simulink model "Fuel_system"  (R2017b)
settings: Solver=ode1  StartTime=0.0  StopTime=inf  FixedStep=0.001  RelTol=1e-3
model workspace (MAT data in the model file):
  sample_time = Simulink.Parameter
  sample_time.DataType = 'auto'
  sample_time.Dimensions = [0 0]
libraries: SIPLib x1
settings Model: Creator=pavel.dushkin  LastModifiedBy=pavel.dushkin
settings DataIOCC: SaveFormat=StructureWithTime  SaveState=on  ReturnWorkspaceOutputs=on
settings OptimizationCC: OptimizeBlockIOStorage=off  BufferReuse=off  GlobalBufferReuse=off  ExpressionFolding=off  LocalBlockOutputs=off  OptimizeDataStoreBuffers=off  BusAssignmentInplaceUpdate=off
settings DebuggingCC: ReadBeforeWriteMsg=DisableAll  WriteAfterWriteMsg=DisableAll  WriteAfterReadMsg=DisableAll  MultiTaskDSMMsg=none
settings ModelReferenceCC: UpdateModelReferenceTargets=IfOutOfDate

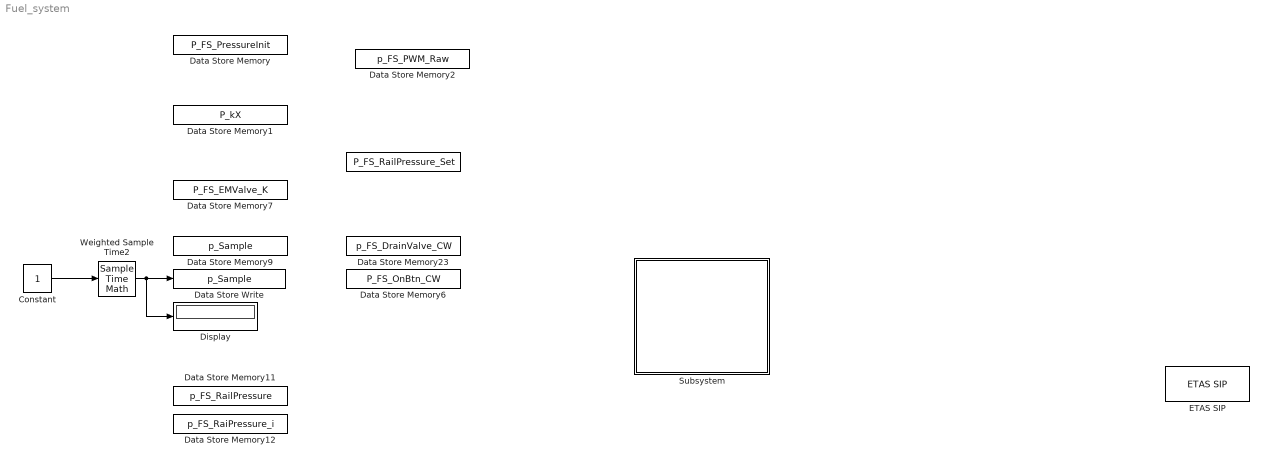
== system Fuel_system ==
  " " : DataStoreMemory  DataStoreName=P_FS_RailPressure_Set  ReadBeforeWriteMsg=warning  WriteAfterWriteMsg=warning  WriteAfterReadMsg=warning  ShowAdditionalParam=off  OutDataTypeStr=double
  Constant : Constant  OutDataTypeStr=double
  Data Store Memory : DataStoreMemory  DataStoreName=P_FS_PressureInit  ReadBeforeWriteMsg=warning  WriteAfterWriteMsg=warning  WriteAfterReadMsg=warning  ShowAdditionalParam=off  OutDataTypeStr=double
  Data Store Memory1 : DataStoreMemory  DataStoreName=P_kX  ReadBeforeWriteMsg=warning  WriteAfterWriteMsg=warning  WriteAfterReadMsg=warning  ShowAdditionalParam=off  OutDataTypeStr=double
  Data Store Memory11 : DataStoreMemory  DataStoreName=p_FS_RailPressure  ReadBeforeWriteMsg=warning  WriteAfterWriteMsg=warning  WriteAfterReadMsg=warning  ShowAdditionalParam=off  OutDataTypeStr=double
  Data Store Memory12 : DataStoreMemory  DataStoreName=p_FS_RaiPressure_i  ReadBeforeWriteMsg=warning  WriteAfterWriteMsg=warning  WriteAfterReadMsg=warning  ShowAdditionalParam=off  OutDataTypeStr=double
  Data Store Memory2 : DataStoreMemory  DataStoreName=p_FS_PWM_Raw  ReadBeforeWriteMsg=warning  WriteAfterWriteMsg=warning  WriteAfterReadMsg=warning  ShowAdditionalParam=off  OutDataTypeStr=double
  Data Store Memory23 : DataStoreMemory  DataStoreName=p_FS_DrainValve_CW  ReadBeforeWriteMsg=warning  WriteAfterWriteMsg=warning  WriteAfterReadMsg=warning  ShowAdditionalParam=off  OutDataTypeStr=double
  Data Store Memory6 : DataStoreMemory  DataStoreName=P_FS_OnBtn_CW  ReadBeforeWriteMsg=warning  WriteAfterWriteMsg=warning  WriteAfterReadMsg=warning  ShowAdditionalParam=off  OutDataTypeStr=double
  Data Store Memory7 : DataStoreMemory  DataStoreName=P_FS_EMValve_K  ReadBeforeWriteMsg=warning  WriteAfterWriteMsg=warning  WriteAfterReadMsg=warning  ShowAdditionalParam=off  OutDataTypeStr=double
  Data Store Memory9 : DataStoreMemory  DataStoreName=p_Sample  ReadBeforeWriteMsg=warning  WriteAfterWriteMsg=warning  WriteAfterReadMsg=warning  ShowAdditionalParam=off  OutDataTypeStr=double
  Data Store Write : DataStoreWrite  DataStoreName=p_Sample
  Display : Display
  ETAS SIP : SIPLib/ETAS SIP
  Subsystem : Subsystem
  Weighted Sample Time2 : SampleTimeMath  TsampMathOp=Ts Only
  wires:
  Weighted Sample Time2/1 -> Display/1, Data Store Write/1
  Constant/1 -> Weighted Sample Time2/1

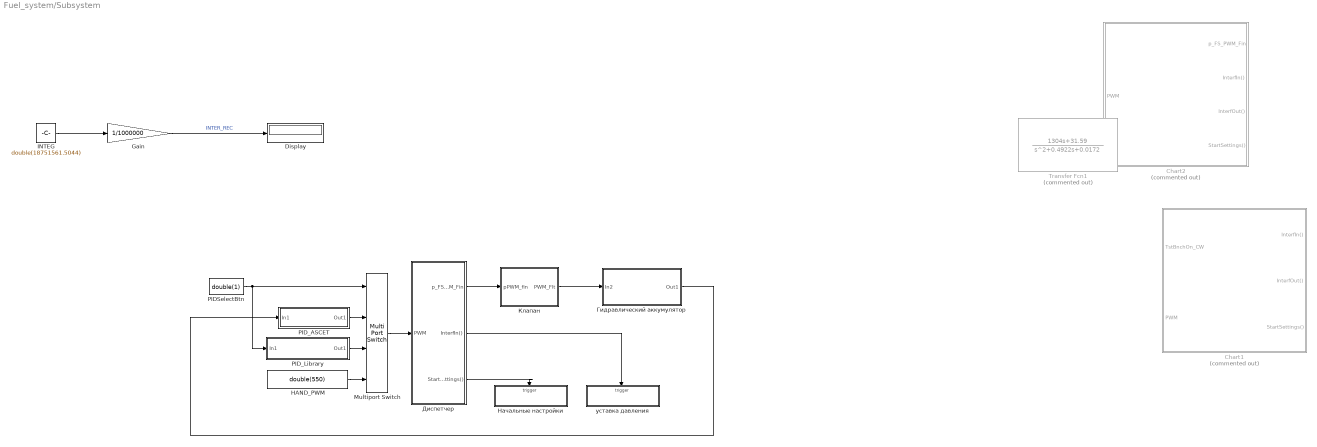
== system Fuel_system/Subsystem ==
  Chart1 : Stateflow chart  Commented=on  TreatAsAtomicUnit=on
  Chart2 : Stateflow chart  Commented=on  TreatAsAtomicUnit=on
  Display : Display
  Gain : Gain  Gain=1/1000000
  HAND_PWM : Constant  Value=double(550)  OutDataTypeStr=single
  INTEG : Constant  Value=double(18751561.5044)
  Multiport Switch : MultiPortSwitch
  PIDSelectBtn : Constant  Value=double(1)  OutDataTypeStr=uint8
  PID_ASCET : Subsystem
  PID_Library : Subsystem
  Transfer Fcn1 : TransferFcn  Commented=on  Numerator=[1304 31.59]  Denominator=[1 0.4922 0.0172]
  Гидравлический аккумулятор : Subsystem
  Диспетчер : Stateflow chart  TreatAsAtomicUnit=on
  Клапан : Subsystem
  Начальные настройки : Subsystem
  уставка давления : Subsystem
  wires:
  PID_ASCET/1(Out1) -> Multiport Switch/2
  HAND_PWM/1 -> Multiport Switch/4
  PID_Library/1(Out1) -> Multiport Switch/3
  PIDSelectBtn/1 -> Multiport Switch/1, PID_Library/1(In1)
  Диспетчер/3(StartSettings()) -> Начальные настройки/Trigger
  Multiport Switch/1 -> Диспетчер/1(PWM)
  Диспетчер/2(InterfIn()) -> уставка давления/Trigger
  Гидравлический аккумулятор/1(Out1) -> PID_ASCET/1(In1)
  INTEG/1 -> Gain/1
  Gain/1 -> Display/1  "INTER_REC"
  Диспетчер/1(p_FS_PWM_Fin) -> Клапан/1(pPWM_fin)
  Клапан/1(PWM_Flt) -> Гидравлический аккумулятор/1(In2)

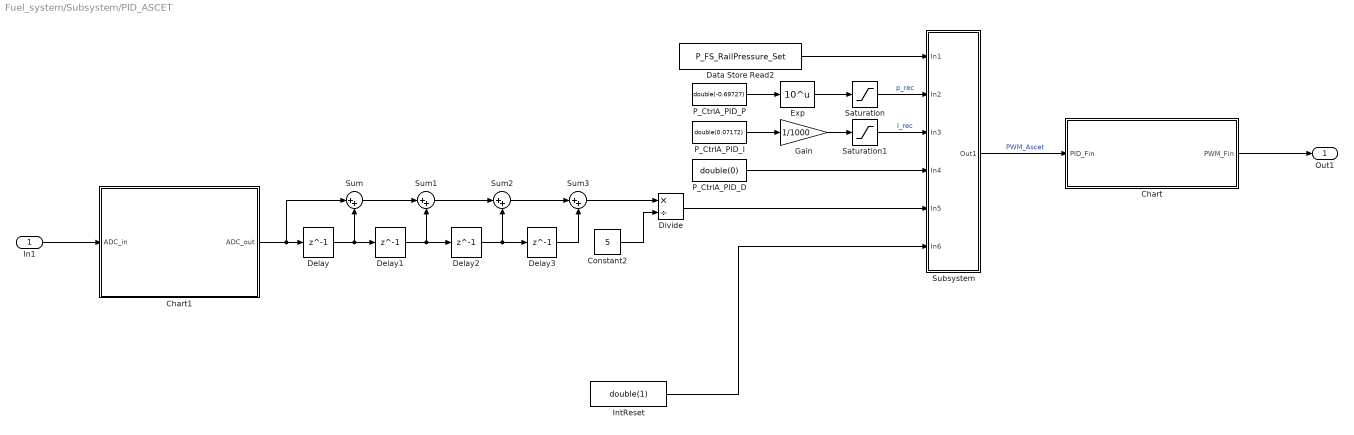
== system Fuel_system/Subsystem/PID_ASCET ==
  In1 : Inport
  Chart : Stateflow chart  TreatAsAtomicUnit=on
  Chart1 : Stateflow chart  TreatAsAtomicUnit=on
  Constant2 : Constant  Value=5
  Data Store Read2 : DataStoreRead  DataStoreName=P_FS_RailPressure_Set
  Delay{,1..3} (4 alike) : Delay  DelayLength=1  InitialCondition=0
  Divide : Product  Inputs=*/  OutDataTypeStr=single
  Exp : Math  Operator=10^u  OutputSignalType=real  SaturateOnIntegerOverflow=on
  Gain : Gain  Gain=1/1000
  IntReset : Constant  Value=double(1)  OutDataTypeStr=single
  P_CtrlA_PID_D : Constant  Value=double(0)  OutDataTypeStr=single
  P_CtrlA_PID_I : Constant  Value=double(0.07172)  OutDataTypeStr=single
  P_CtrlA_PID_P : Constant  Value=double(-0.69727)  OutDataTypeStr=single
  Saturation : Saturate  UpperLimit=inf  LowerLimit=0
  Saturation1 : Saturate  UpperLimit=inf  LowerLimit=0.01/1000
  Subsystem : Subsystem
  Sum{,1..3} (4 alike) : Sum  Inputs=|++
  Out1 : Outport
  wires:
  P_CtrlA_PID_D/1 -> Subsystem/4(In4)
  P_CtrlA_PID_P/1 -> Exp/1
  P_CtrlA_PID_I/1 -> Gain/1
  Subsystem/1(Out1) -> Chart/1(PID_Fin)  "PWM_Ascet"
  Data Store Read2/1 -> Subsystem/1(In1)
  Divide/1 -> Subsystem/5(In5)
  IntReset/1 -> Subsystem/6(In6)
  Chart1/1(ADC_out) -> Sum/1, Delay/1
  Delay/1 -> Sum/2, Delay1/1
  Delay1/1 -> Sum1/2, Delay2/1
  Delay2/1 -> Sum2/2, Delay3/1
  Delay3/1 -> Sum3/2
  Sum/1 -> Sum1/1
  Sum1/1 -> Sum2/1
  Sum2/1 -> Sum3/1
  Sum3/1 -> Divide/1
  Constant2/1 -> Divide/2
  Chart/1(PWM_Fin) -> Out1/1
  Gain/1 -> Saturation1/1
  Exp/1 -> Saturation/1
  In1/1 -> Chart1/1(ADC_in)
  Saturation/1 -> Subsystem/2(In2)  "p_rec"
  Saturation1/1 -> Subsystem/3(In3)  "I_rec"

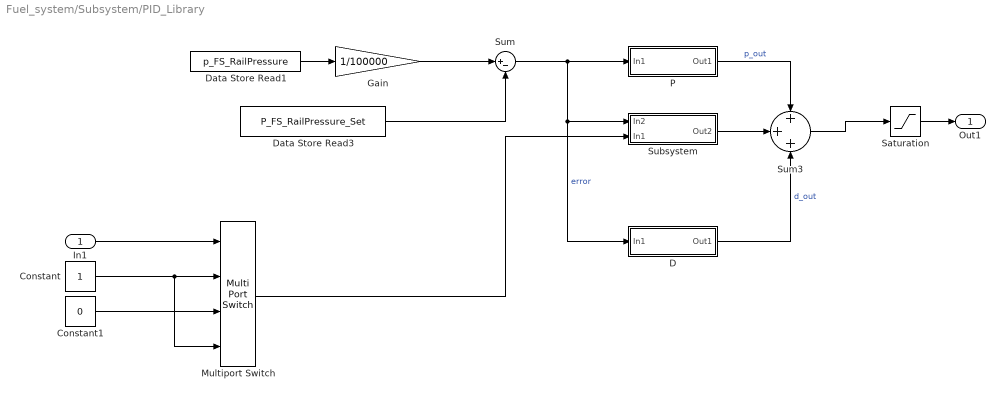
== system Fuel_system/Subsystem/PID_Library ==
  In1 : Inport
  Constant : Constant
  Constant1 : Constant  Value=0
  D : Subsystem
  Data Store Read1 : DataStoreRead  DataStoreName=p_FS_RailPressure
  Data Store Read3 : DataStoreRead  DataStoreName=P_FS_RailPressure_Set
  Gain : Gain  Gain=1/100000
  Multiport Switch : MultiPortSwitch
  P : Subsystem
  Saturation : Saturate  UpperLimit=50  LowerLimit=30
  Subsystem : Subsystem
  Sum : Sum  Inputs=|+-
  Sum3 : Sum  Inputs=+++
  Out1 : Outport
  wires:
  Sum3/1 -> Saturation/1
  P/1(Out1) -> Sum3/1  "p_out"
  Data Store Read1/1 -> Gain/1
  Saturation/1 -> Out1/1
  Sum/1 -> Subsystem/1(In2), D/1(In1), P/1(In1)  "error"
  D/1(Out1) -> Sum3/3  "d_out"
  Subsystem/1(Out2) -> Sum3/2
  In1/1 -> Multiport Switch/1
  Constant/1 -> Multiport Switch/4, Multiport Switch/2
  Multiport Switch/1 -> Subsystem/2(In1)
  Constant1/1 -> Multiport Switch/3
  Data Store Read3/1 -> Sum/2
  Gain/1 -> Sum/1

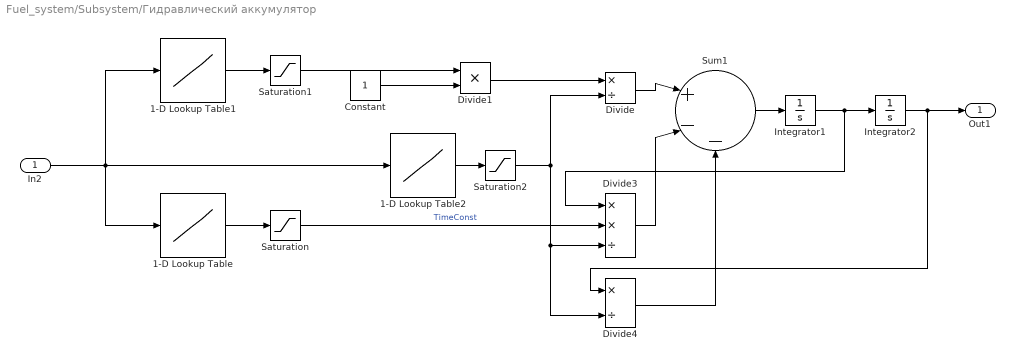
== system Fuel_system/Subsystem/Гидравлический аккумулятор ==
  In2 : Inport
  1-D Lookup Table : Lookup_n-D  NumberOfTableDimensions=1  BreakpointsForDimension1=[100 450 500 550]  Table=[0.03 0.03 1.55 9]  InternalRulePriority=Speed  RndMeth=Simplest  InputSameDT=on
  1-D Lookup Table1 : Lookup_n-D  NumberOfTableDimensions=1  BreakpointsForDimension1=[100 450 500 550]  Table=[3500 2500 1950 925]  InternalRulePriority=Speed  RndMeth=Simplest  InputSameDT=on
  1-D Lookup Table2 : Lookup_n-D  NumberOfTableDimensions=1  BreakpointsForDimension1=[100 450 500 550]  Table=[0.2 0.5 1 1]  InternalRulePriority=Speed  RndMeth=Simplest  InputSameDT=on
  Constant : Constant
  Divide : Product  Inputs=*/  OutDataTypeStr=single
  Divide1 : Product  Inputs=**  OutDataTypeStr=single
  Divide3 : Product  Inputs=**/
  Divide4 : Product  Inputs=*/
  Integrator1 : Integrator
  Integrator2 : Integrator
  Saturation : Saturate  UpperLimit=inf  LowerLimit=0.01
  Saturation1 : Saturate  UpperLimit=5000  LowerLimit=0
  Saturation2 : Saturate  UpperLimit=inf  LowerLimit=0.1
  Sum1 : Sum  Inputs=|+--  AccumDataTypeStr=single
  Out1 : Outport
  wires:
  Integrator2/1 -> Out1/1, Divide4/1
  Divide/1 -> Sum1/1
  Sum1/1 -> Integrator1/1
  Integrator1/1 -> Divide3/1, Integrator2/1
  1-D Lookup Table2/1 -> Saturation2/1
  Divide4/1 -> Sum1/3
  Divide3/1 -> Sum1/2
  1-D Lookup Table/1 -> Saturation/1
  1-D Lookup Table1/1 -> Saturation1/1
  Constant/1 -> Divide1/2
  Saturation1/1 -> Divide1/1
  Saturation/1 -> Divide3/2  "TimeConst"
  In2/1 -> 1-D Lookup Table2/1, 1-D Lookup Table/1, 1-D Lookup Table1/1
  Saturation2/1 -> Divide/2, Divide4/2, Divide3/3
  Divide1/1 -> Divide/1

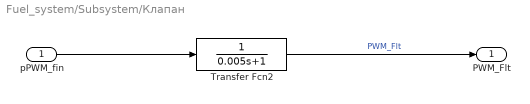
== system Fuel_system/Subsystem/Клапан ==
  pPWM_fin : Inport
  Transfer Fcn2 : TransferFcn  Denominator=[0.005 1]
  PWM_Flt : Outport
  wires:
  pPWM_fin/1 -> Transfer Fcn2/1
  Transfer Fcn2/1 -> PWM_Flt/1  "PWM_Flt"

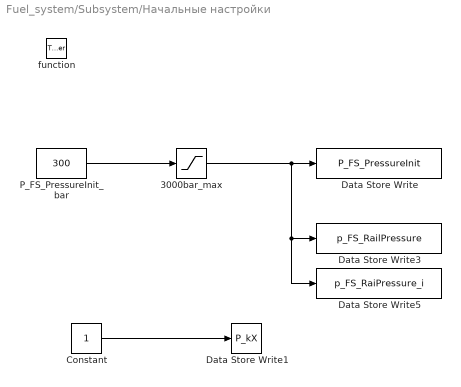
== system Fuel_system/Subsystem/Начальные настройки ==
  function : TriggerPort  TriggerType=function-call  VariantControl=(inherit)
  3000bar_max : Saturate  UpperLimit=3000  LowerLimit=0
  Constant : Constant
  Data Store Write : DataStoreWrite  DataStoreName=P_FS_PressureInit
  Data Store Write1 : DataStoreWrite  DataStoreName=P_kX
  Data Store Write3 : DataStoreWrite  DataStoreName=p_FS_RailPressure
  Data Store Write5 : DataStoreWrite  DataStoreName=p_FS_RaiPressure_i
  P_FS_PressureInit_bar : Constant  Value=300  OutDataTypeStr=double
  wires:
  3000bar_max/1 -> Data Store Write5/1, Data Store Write3/1, Data Store Write/1
  P_FS_PressureInit_bar/1 -> 3000bar_max/1
  Constant/1 -> Data Store Write1/1

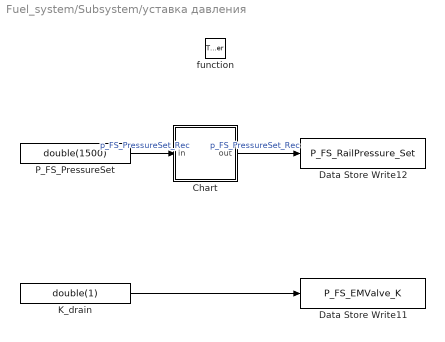
== system Fuel_system/Subsystem/уставка давления ==
  function : TriggerPort  TriggerType=function-call  VariantControl=(inherit)
  Chart : Stateflow chart  TreatAsAtomicUnit=on
  Data Store Write11 : DataStoreWrite  DataStoreName=P_FS_EMValve_K
  Data Store Write12 : DataStoreWrite  DataStoreName=P_FS_RailPressure_Set
  K_drain : Constant  Value=double(1)  OutDataTypeStr=double
  P_FS_PressureSet : Constant  Value=double(1500)  OutDataTypeStr=double
  wires:
  K_drain/1 -> Data Store Write11/1
  Chart/1(out) -> Data Store Write12/1  "p_FS_PressureSet_Rec"
  P_FS_PressureSet/1 -> Chart/1(in)  "p_FS_PressureSet_Rec"

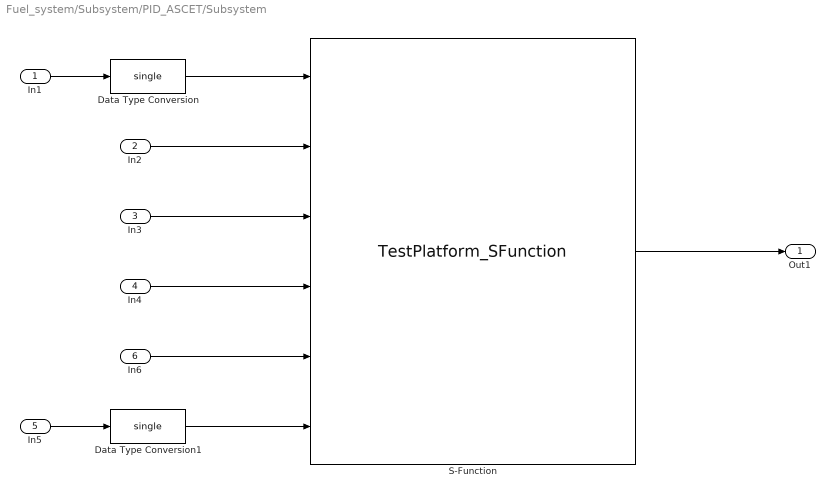
== system Fuel_system/Subsystem/PID_ASCET/Subsystem ==
  In1 : Inport
  In2 : Inport  Port=2
  In3 : Inport  Port=3
  In4 : Inport  Port=4
  In5 : Inport  Port=5
  In6 : Inport  Port=6
  Data Type Conversion : DataTypeConversion  OutDataTypeStr=single
  Data Type Conversion1 : DataTypeConversion  OutDataTypeStr=single
  S-Function : S-Function  InitFcn=clear TestPlatform_SFunction  FunctionName=TestPlatform_SFunction  SFunctionDeploymentMode=off  EnableBusSupport=off
      mask Display:
      | disp('TestPlatform_SFunction')
      | port_label('output',1,'components.InpOut.PWM')
      | port_label('input',1,'components.PID.PressSet')
      | port_label('input',2,'components.PID.qP')
      | port_label('input',3,'components.PID.qI')
      | port_label('input',4,'components.PID.qD')
      | port_label('input',5,'components.PID.I_reset')
      | port_label('input',6,'components.InpOut.MeasuredPressure')
  Out1 : Outport
  wires:
  In1/1 -> Data Type Conversion/1
  In5/1 -> Data Type Conversion1/1
  Data Type Conversion/1 -> S-Function/1
  In2/1 -> S-Function/2
  In3/1 -> S-Function/3
  In4/1 -> S-Function/4
  In6/1 -> S-Function/5
  Data Type Conversion1/1 -> S-Function/6
  S-Function/1 -> Out1/1

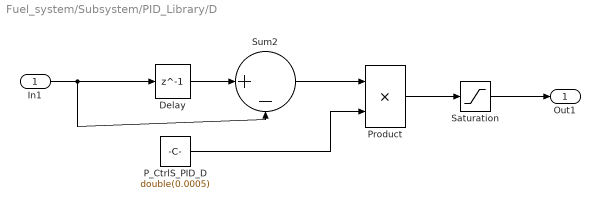
== system Fuel_system/Subsystem/PID_Library/D ==
  In1 : Inport
  Delay : Delay  DelayLength=1
  P_CtrlS_PID_D : Constant  Value=double(0.0005)
  Product : Product
  Saturation : Saturate  UpperLimit=100  LowerLimit=-100
  Sum2 : Sum  Inputs=|+-
  Out1 : Outport
  wires:
  Sum2/1 -> Product/1
  Saturation/1 -> Out1/1
  In1/1 -> Sum2/2, Delay/1
  P_CtrlS_PID_D/1 -> Product/2
  Product/1 -> Saturation/1
  Delay/1 -> Sum2/1

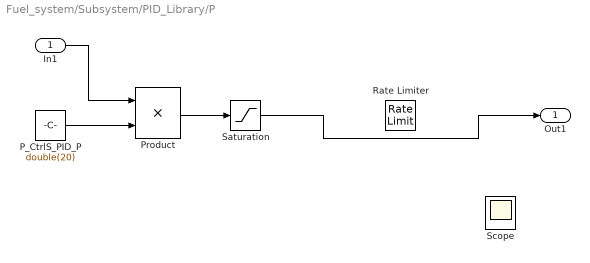
== system Fuel_system/Subsystem/PID_Library/P ==
  In1 : Inport
  P_CtrlS_PID_P : Constant  Value=double(20)
  Product : Product
  Rate Limiter : RateLimiter  RisingSlewLimit=5  FallingSlewLimit=-5  SampleTimeMode=inherited
  Saturation : Saturate  UpperLimit=100  LowerLimit=0
  Scope : Scope  NumInputPorts=2
  Out1 : Outport
  wires:
  In1/1 -> Product/1
  Product/1 -> Saturation/1
  P_CtrlS_PID_P/1 -> Product/2
  Saturation/1 -> Out1/1

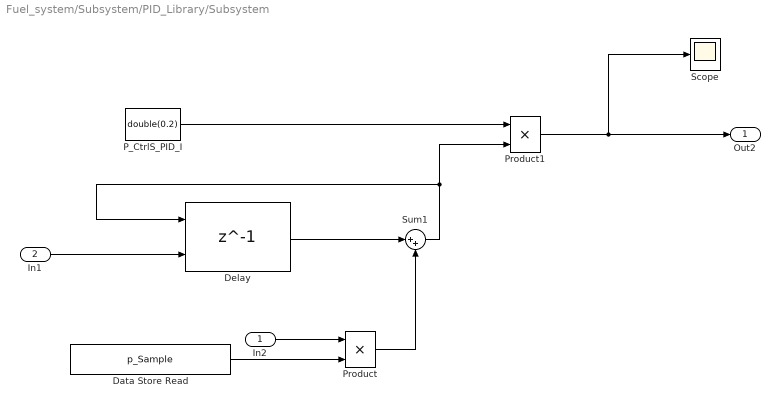
== system Fuel_system/Subsystem/PID_Library/Subsystem ==
  In2 : Inport
  In1 : Inport  Port=2
  Data Store Read : DataStoreRead  DataStoreName=p_Sample
  Delay : Delay  DelayLength=1  ExternalReset=Level
      settings: InputPortMap=u0,r5
  P_CtrlS_PID_I : Constant  Value=double(0.2)
  Product : Product
  Product1 : Product
  Scope : Scope
  Sum1 : Sum  Inputs=|++
  Out2 : Outport
  wires:
  Data Store Read/1 -> Product/2
  P_CtrlS_PID_I/1 -> Product1/1
  Product1/1 -> Out2/1, Scope/1
  In2/1 -> Product/1
  Sum1/1 -> Delay/1, Product1/2
  Product/1 -> Sum1/2
  Delay/1 -> Sum1/1
  In1/1 -> Delay/2

== stateflow chart Fuel_system/Subsystem/уставка давления/Chart ==
  (default) -> (junction 3) : {out=(in-out)*0.35+out;}
  data: in input; out output =0

== stateflow chart Fuel_system/Subsystem/PID_ASCET/Chart ==
  (default) -> (junction 12) : {PWM_Fin=PID_Fin*(-1.023)+1023}
  (junction 12) -> (junction 20) [order 3] : [PWM_Fin>=920]{PWM_Fin=920}
  (junction 12) -> (junction 21) [order 2] : [PWM_Fin<=0]{PWM_Fin=0}
  (junction 21) -> (junction 22)
  (junction 20) -> (junction 22)
  (junction 12) -> (junction 22) [order 1] : [(PWM_Fin>0)&(PWM_Fin<920)]
  data: PID_Fin input; PWM_Fin output

== stateflow chart Fuel_system/Subsystem/Диспетчер ==
  (default) -> (junction 8) : [start_fl==0]
  (junction 8) -> (junction 10) [order 2] : {StartSettings;
      | start_fl=1;}
  (junction 8) -> (junction 50) [order 1] : {InterfIn;}
  (junction 50) -> (junction 59) [order 2] : {PWM_count++;}
  (junction 59) -> (junction 56)
  (junction 50) -> (junction 56) [order 1] : [PWM_count>=40]
      | {
      | p_FS_PWM_Fin=PWM;
      | PWM_count=0;
      | }
  (junction 56) -> (junction 18) : {InterfOut;}
  data: start_fl local double =0; P_kX data_store_memory; p_FS_RailPressure data_store_memory; P_FS_EMValve_K data_store_memory; drain_open local double; PWM input double; PWM_count local double; p_FS_PWM_Fin output double; PWM_Temp local double
  events: InterfIn output FUNCTION_CALL_EVENT; StartSettings output FUNCTION_CALL_EVENT

== stateflow chart Fuel_system/Subsystem/Chart1 ==
  (default) -> (junction 8) : [start_fl==0]
  (junction 8) -> (junction 10) [order 2] : {StartSettings;
      | start_fl=1;}
  (junction 8) -> (junction 28) [order 1] : {InterfIn;}
  (junction 28) -> (junction 30) [order 2] : %{P_kX=1-(p_FS_RailPressure-750)*P_FS_EMValve_K;
      | %drain_open=1;}
  (junction 30) -> (junction 45) [order 2] : %{P_kX=0;}
  (junction 45) -> (junction 32)
  (junction 30) -> (junction 32) [order 1] : %[P_kX>0]
  (junction 28) -> (junction 32) [order 1] : %[(p_FS_RailPressure<=1950)&(drain_open==0)]
      | %{P_kX=1;}
  (junction 32) -> (junction 50) [order 2]
  (junction 32) -> (junction 50) [order 1] : %[p_FS_RailPressure<750]
      | %{drain_open=0;}
  (junction 50) -> (junction 59) [order 2] : {PWM_count++;}
  (junction 59) -> (junction 56)
  (junction 50) -> (junction 56) [order 1] : [PWM_count>=20]
      | {
      | p_FS_PWM_Fin=PWM;
      | PWM_count=0;
      | }
  (junction 56) -> (junction 18) : {InterfOut;}
  data: TstBnchOn_CW input; start_fl local double =0; P_kX data_store_memory; p_FS_RailPressure data_store_memory; P_FS_EMValve_K data_store_memory; drain_open local double; PWM input double; p_FS_PWM_Fin data_store_memory; PWM_count local double
  events: InterfIn output FUNCTION_CALL_EVENT; InterfOut output FUNCTION_CALL_EVENT; StartSettings output FUNCTION_CALL_EVENT

== stateflow chart Fuel_system/Subsystem/Chart2 ==
  (default) -> (junction 8) : [start_fl==0]
  (junction 8) -> (junction 10) [order 2] : {StartSettings;
      | start_fl=1;}
  (junction 8) -> (junction 66) [order 1] : {InterfIn;}
  (junction 66) -> (junction 67) : {PWM_Temp=-1.4286*PWM + 785.71;}
  (junction 67) -> (junction 70) [order 2] : [PWM_Temp<=0]{PWM_Temp=0;}
  (junction 67) -> (junction 75) [order 3] : {PWM_Temp=120;}
  (junction 70) -> (junction 50)
  (junction 75) -> (junction 50)
  (junction 67) -> (junction 50) [order 1] : [(PWM_Temp>0)&(PWM_Temp<120)]
  (junction 50) -> (junction 59) [order 2] : {PWM_count++;}
  (junction 59) -> (junction 56)
  (junction 50) -> (junction 56) [order 1] : [PWM_count>=40]
      | {
      | p_FS_PWM_Fin=PWM_Temp/100;
      | PWM_count=0;
      | }
  (junction 56) -> (junction 18) : {InterfOut;}
  data: start_fl local double =0; P_kX data_store_memory; p_FS_RailPressure data_store_memory; P_FS_EMValve_K data_store_memory; drain_open local double; PWM input double; PWM_count local double; p_FS_PWM_Fin output double; PWM_Temp local double
  events: InterfIn output FUNCTION_CALL_EVENT; InterfOut output FUNCTION_CALL_EVENT; StartSettings output FUNCTION_CALL_EVENT

== stateflow chart Fuel_system/Subsystem/PID_ASCET/Chart1 ==
  (default) -> (junction 2) [order 1]
  (junction 2) -> (junction 7) [order 2] : {ADC_count = ADC_count + 1;}
  (default) -> (junction 1) [order 2]
  (junction 2) -> (junction 1) [order 1] : [ADC_count>=5]
      | {
      | ADC_out=ADC_in;
      | ADC_count=0;
      | }
  data: ADC_out output; ADC_in input; ADC_count local =0
